simulink library "FIREven"  (R2022b)
settings: Solver=VariableStepAuto  StartTime=0.0  StopTime=10.0  RelTol=1e-3
settings Model: Creator=jb10849  LastModifiedBy=kl13806
settings SolverCC: AlgebraicLoopSolver=TrustRegion
settings DebuggingCC: UnconnectedInputMsg=warning  UnconnectedOutputMsg=warning  UnconnectedLineMsg=warning  SFMachineParentedDataDiag=warning  ArithmeticOperatorsInVariantConditions=warning
settings ModelReferenceCC: EnableRefExpFcnMdlSchedulingChecks=on
settings SFSimCC: SimUseLocalCustomCode=off  CustomCodeUndefinedFunction=UseInterfaceOnly
settings RTWCC: RTWUseLocalCustomCode=off  DLArmComputeVersion=19.05
settings CodeAppCC: StateflowObjectComments=on

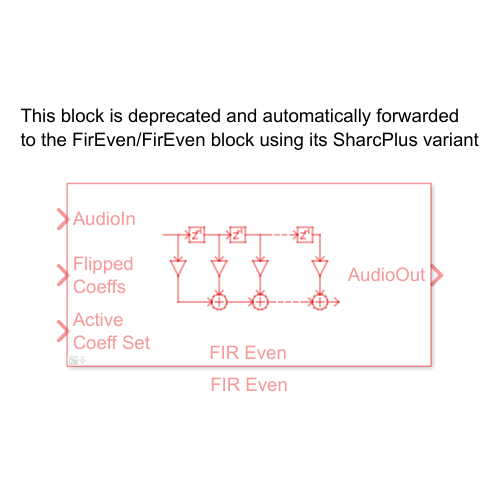
[thumbnail: Simulink's stored preview of the top-level diagram]
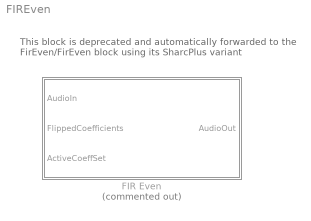
== system FIREven ==
  note: This block is deprecated and automatically forwarded
      | to the FirEven/FirEven block using its SharcPlus variant
  FIR Even : Subsystem  Commented=on  mask(Bose FIR Even){}
      mask help: Bose FIR Even: Finite Impulse Response filter
      mask Display:
      | [path,w,h] = IconFIR_Mask();
      | 
      | port_label('input', 1, 'AudioIn');
      | port_label('input', 2, sprintf('Flipped\nCoeffs'));
      | port_label('input', 3, sprintf('Active\nCoeff Set'));
      | port_label('output', 1, 'AudioOut');
      | 
      | % work in pixels since the icon does not scale
      | pos = get(gcbh,'position');
      | bw = pos(3) - pos(1);
      | bh = pos(4) - pos(2);
      | 
      | % Draw centered icon
      | xAdj = bw/2 - w/2;
      | yAdj = bh/2 - h/2 + 4;
      | for i=1:length(path)
      | %     patch(path(i).x+xAdj, path(i).y+yAdj, path(i).rgb);
      |     plot(path(i).x+xAdj, path(i).y+yAdj);
      | end
      | 
      | % Anchor the corners of the coordinate system
      | patch(0,0,[1 1 1]);
      | patch(bw,bh,[1 1 1]);
      | 
      | % Display some text
      | text(bw/2, 1,'FIR Even', ...
      |     'horizontalAlignment','center', ...
      |     'VerticalAlignment','bottom');

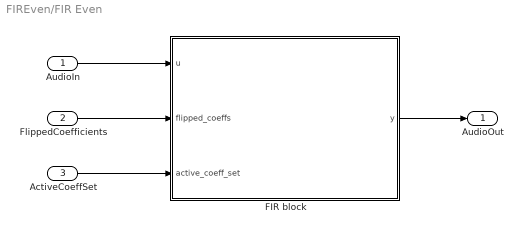
== system FIREven/FIR Even ==
  AudioIn : Inport
  FlippedCoefficients : Inport  Port=2
  ActiveCoeffSet : Inport  Port=3
  "FIR block " : MATLAB Function  TreatAsAtomicUnit=on
  AudioOut : Outport  VectorParamsAs1DForOutWhenUnconnected=off
  wires:
  "FIR block "/1(y) -> AudioOut/1
  AudioIn/1 -> "FIR block "/1(u)
  FlippedCoefficients/1 -> "FIR block "/2(flipped_coeffs)
  ActiveCoeffSet/1 -> "FIR block "/3(active_coeff_set)

== matlab function FIREven/FIR Even/FIR block  ==
  data: u input; y output; flipped_coeffs input single; active_coeff_set input
function y = fir_even_filter(u, flipped_coeffs, active_coeff_set)

% Extract configuration information from inputs
[taps, ~] = size(flipped_coeffs);
[frame_size, num_channels] = size(u);

% Initialize state variables to zero
persistent states;
if isempty(states)
    states = single(zeros(taps + 2, num_channels));
end
% Initialize state index to zero
persistent state_index;
if isempty(state_index)
    state_index = uint32(0);
end

% Set correct data types
filter_length = uint32(taps);
frame_size = uint32(frame_size);
num_channels = uint32(num_channels);
active_coeff_set = uint32(active_coeff_set);
% Invoking the fir_even function
y = fir_even(u, frame_size, num_channels, states, filter_length, state_index, active_coeff_set, flipped_coeffs);


function y = fir_even(u, framesize, numChannels, states, filterLength, stateIndex, activeCoeffSet, coeffs)
% If target == codegen, generate warning if no CRL found
coder.replace('-warnifnoreplacement');

% If running simulation, just use filter()
% Matlab function takes unflipped coeffs, so coeffs needs to be flipped
a = 1;
b = flipud(coeffs);
[taps, ~] = size(b);

persistent zi;
if isempty(zi)
    zi = single(zeros(taps - 1, numChannels));
end

y = single(zeros(size(u)));
for i = 1:numChannels
    % Get input, filter coeffs and state for this channel
    u0 = u(:, i);
    filterIdx = activeCoeffSet(i) + 1; % add 1 for Matlab indexing
    coeff = b(:, filterIdx);
    state = zi(:, i);
    
    % Compute output samples and state
    [y0, state] = filter(coeff, a, u0, state);
    y(:, i) = y0;
    
    % Save state
    zi(:, i) = state;
end
